simulink model "sim"  (R2020a)
settings: Solver=ode45  StartTime=0.0  StopTime=200  RelTol=1e-3  EnableMultiTasking=on
settings Model: Creator=CD  LastModifiedBy=user
settings DataIOCC: ExternalInput=[t u]  LimitDataPoints=on  SaveFormat=Array  ReturnWorkspaceOutputs=off
settings OptimizationCC: LifeSpan=inf
settings DebuggingCC: UnderspecifiedInitializationDetection=Classic  MergeDetectMultiDrivingBlocksExec=none  SolverPrmCheckMsg=warning  SFUnexpectedBacktrackingDiag=warning  SFNoUnconditionalDefaultTransitionDiag=warning  SFExecutionAtInitializationDiag=none  ArithmeticOperatorsInVariantConditions=warning
settings HardwareCC: ProdBitPerPointer=32  ProdBitPerSizeT=32  ProdBitPerPtrDiffT=32  ProdLargestAtomicFloat=None  ProdIntDivRoundTo=Undefined  ProdEndianess=Unspecified  ProdWordSize=32  ProdHWDeviceType=32-bit Generic
settings ModelReferenceCC: PropagateSignalLabelsOutOfModel=off
settings SFSimCC: SimUseLocalCustomCode=off  CustomCodeUndefinedFunction=UseInterfaceOnly
settings RTWCC: RTWUseLocalCustomCode=off
settings CodeAppCC: StateflowObjectComments=on
settings GRTTargetCC: TargetLangStandard=C89/C90 (ANSI)
settings ConfigComp: CovMetricSettings=dw  CovHtmlReporting=on  CovSaveCumulativeToWorkspaceVar=on  CovSaveSingleToWorkspaceVar=on  CovExternalEMLEnable=off

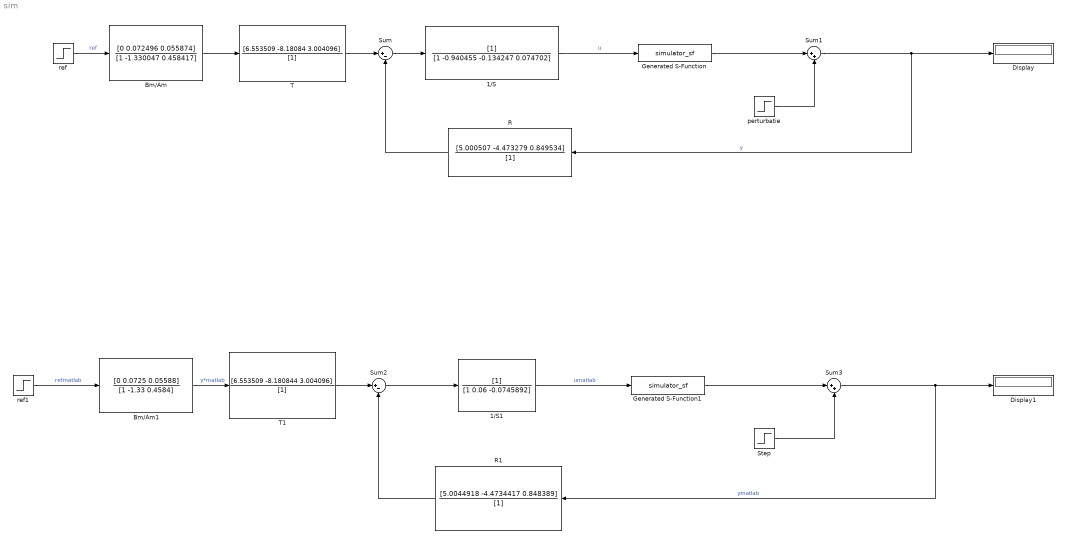
== system sim ==
  1/S : DiscreteFilter  Denominator=[1 -0.940455 -0.134247 0.074702]  SampleTime=0.6
  1/S1 : DiscreteFilter  Denominator=[1 0.06 -0.0745892]  SampleTime=0.6
  Bm/Am : DiscreteFilter  Numerator=[0 0.072496 0.055874]  Denominator=[1 -1.330047 0.458417]  SampleTime=0.6
  Bm/Am1 : DiscreteFilter  Numerator=[0 0.0725 0.05588]  Denominator=[1 -1.33 0.4584]  SampleTime=0.6
  Display : Display
  Display1 : Display
  Generated S-Function : S-Function  FunctionName=simulator_sf  SFunctionModules=""  SFunctionDeploymentMode=off  EnableBusSupport=off  mask{rtw_sf_name=simulator_sf, showVar=off}
      mask prompts: rtw_sf_name "Simulink:masks:GenSFuncName_MP"; showVar "Simulink:masks:GenSFuncShowModuleList_MP"
      mask help: Simulink:masks:GenSFuncDesc_MD
      mask init:
      | displist = '';
      | if ~strcmp(get_param(gcb, 'FunctionName'), rtw_sf_name);
      |   set_param(gcb, 'FunctionName', rtw_sf_name);
      | end
      | % Check if we are generating code
      | rtw_mode = false;
      | if strcmpi(get_param(bdroot(gcb),'SimulationStatus'),'Initializing')
      | 	rtw_mode = strcmpi(get_param(bdroot(gcb),'BuildingRTWCode'),'on') && ...
      | 		~strcmpi(get_param(bdroot(gcb),'TargetStyle'),'SimulationTarget');
      | end
      | if showVar || rtw_mode
      | 	if exist('rtwsfunc') == 2 | exist('rtwsfunc') == 6
      | 		tmplist = rtwsfunc(rtw_sf_name,gcb);
      | 		tmplist = DAStudio.message('Simulink:masks:GenSFuncListOfModules_IC', tmplist);
      | 	elseif showVar
      | 		tmplist1 = DAStudio.message('Simulink:masks:GenSFuncListOfModules_IC', '');
      |         tmplist2 = DAStudio.message('Simulink:masks:GenSFuncNotLicensed_IC');
      |         tmplist = [tmplist1 tmplist2];
      |  	end
      | end
      | if showVar
      |   displist = tmplist;
      | end
      settings: CopyFcn=|
      | if ~strcmp(get_param(gcb,'Linkstatus'),'none') && ...
      | ~strcmp(get_param(gcb,'Linkstatus'),'implicit')
      |   set_param(gcb,'LinkStatus','none');
      | end
      mask Help: eval('feval(''rtwprivate'',''rtwhelpview'',''rtw_sfcn_block'')');
      mask Display:
      | port_label('input',1,'Commande');
      | port_label('output',1,'Sortie');
  Generated S-Function1 : S-Function  FunctionName=simulator_sf  SFunctionModules=""  SFunctionDeploymentMode=off  EnableBusSupport=off  mask{rtw_sf_name=simulator_sf, showVar=off}
      mask prompts: rtw_sf_name "Simulink:masks:GenSFuncName_MP"; showVar "Simulink:masks:GenSFuncShowModuleList_MP"
      mask help: Simulink:masks:GenSFuncDesc_MD
      mask init: same as sim/Generated S-Function
      settings: CopyFcn=|
      | if ~strcmp(get_param(gcb,'Linkstatus'),'none') && ...
      | ~strcmp(get_param(gcb,'Linkstatus'),'implicit')
      |   set_param(gcb,'LinkStatus','none');
      | end
      mask Help: eval('feval(''rtwprivate'',''rtwhelpview'',''rtw_sfcn_block'')');
      mask Display:
      | port_label('input',1,'Commande');
      | port_label('output',1,'Sortie');
  R : DiscreteFilter  Numerator=[5.000507 -4.473279 0.849534]  Denominator=[1]  SampleTime=0.6
  R1 : DiscreteFilter  Numerator=[5.0044918 -4.4734417 0.848389]  Denominator=[1]  SampleTime=0.6
  Step : Step  Time=50  After=1.5  SampleTime=0.6
  Sum : Sum  Inputs=|+-
  Sum1 : Sum  Inputs=|++
  Sum2 : Sum  Inputs=|+-
  Sum3 : Sum  Inputs=|++
  T : DiscreteFilter  Numerator=[6.553509 -8.18084 3.004096]  Denominator=[1]  SampleTime=0.6
  T1 : DiscreteFilter  Numerator=[6.553509 -8.180844 3.004096]  Denominator=[1]  SampleTime=0.6
  perturbatie : Step  Time=60  After=4.5  SampleTime=0.6
  ref : Step  Time=0  After=6  SampleTime=0.6
  ref1 : Step  Time=0  After=6  SampleTime=0.6
  wires:
  Sum1/1 -> Display/1, R/1  "y"
  perturbatie/1 -> Sum1/2
  R/1 -> Sum/2
  1/S/1 -> Generated S-Function/1  "u"
  Sum/1 -> 1/S/1
  Bm/Am/1 -> T/1
  T/1 -> Sum/1
  ref/1 -> Bm/Am/1  "ref"
  Generated S-Function/1 -> Sum1/1
  ref1/1 -> Bm/Am1/1  "refmatlab"
  Step/1 -> Sum3/2
  Generated S-Function1/1 -> Sum3/1
  Sum3/1 -> R1/1, Display1/1  "ymatlab"
  T1/1 -> Sum2/1
  Sum2/1 -> 1/S1/1
  Bm/Am1/1 -> T1/1  "y*matlab"
  R1/1 -> Sum2/2
  1/S1/1 -> Generated S-Function1/1  "umatlab"
